simulink model "TL1_cs"  (R2019a)
settings: Solver=FixedStepDiscrete  StartTime=0.0  StopTime=40  FixedStep=1/300  RelTol=1e-3
PreLoadFcn:
  | mbxruntime.callbacks.PreLoadFcn(bdroot);
  | check_NUTS_defined
  | model_closed = 0;
  | assignin('base',['model_closed_' bdroot],false);
PostLoadFcn:
  | mbxruntime.callbacks.PostLoadFcn(bdroot);
InitFcn:
  | mbxruntime.callbacks.InitFcn(bdroot);
StartFcn:
  | mbxruntime.callbacks.StartFcn(bdroot);
StopFcn:
  | mbxruntime.callbacks.StopFcn(bdroot);;
  | 
model workspace: external: MAT-File .\TL1_cs_hws.mat (data not in the file)
undefined symbols (not defined in the file): AngularVelocity, Clock_, Data, Data_SL_Info, DiscIntNeverNeededParam, Encoding, Encoding_SL_Info, Header, Height, InitImageOutputDir, LinearAcceleration, mbxruntime, Orientation, Pose, Poses, Poses_SL_Info, Position, Step, tabledata, Twist, Width
libraries: robotlib x24, simulink_extras x16, PreScanSimulinkLibrary x4, dspindex x4, robotcorelib x2, visionconversions x2, visionsinks x2, sharedtransform x1
(part 3 of 4)

== system TL1_cs/BMW_X5_SUV_1/Subsystem2 ==
  In1 : Inport
  In2 : Inport  Port=2
  In3 : Inport  Port=3
  In4 : Inport  Port=4
  In5 : Inport  Port=5
  Matrix Concatenate5 : Concatenate  NumInputs=4  Mode=Multidimensional array  ConcatenateDimension=2
  Reshape{1..4} (4 alike) : Reshape
  Rotate over Z : Subsystem
  Spherical to cartesian : Subsystem
  Out1 : Outport
  wires:
  In5/1 -> Reshape3/1
  Reshape4/1 -> Spherical to cartesian/1(In1)
  In1/1 -> Rotate over Z/1(In1)
  Reshape1/1 -> Spherical to cartesian/2(In2)
  Spherical to cartesian/1(Out1) -> Rotate over Z/2(In2)
  Reshape2/1 -> Spherical to cartesian/3(In3)
  Spherical to cartesian/2(Out2) -> Rotate over Z/3(In3)
  In3/1 -> Reshape1/1
  Rotate over Z/2(Out2) -> Matrix Concatenate5/2
  Spherical to cartesian/3(Out3) -> Matrix Concatenate5/3
  Reshape3/1 -> Matrix Concatenate5/4
  Rotate over Z/1(Out1) -> Matrix Concatenate5/1
  Matrix Concatenate5/1 -> Out1/1
  In2/1 -> Reshape4/1
  In4/1 -> Reshape2/1

== system TL1_cs/BMW_X5_SUV_1/Subsystem3 ==
  In1 : Inport
  In2 : Inport  Port=2
  In3 : Inport  Port=3
  In4 : Inport  Port=4
  In5 : Inport  Port=5
  Matrix Concatenate5 : Concatenate  NumInputs=4  Mode=Multidimensional array  ConcatenateDimension=2
  Reshape{1..4} (4 alike) : Reshape
  Rotate over Z : Subsystem
  Spherical to cartesian : Subsystem
  Out1 : Outport
  wires:
  In5/1 -> Reshape3/1
  Reshape4/1 -> Spherical to cartesian/1(In1)
  In1/1 -> Rotate over Z/1(In1)
  Reshape1/1 -> Spherical to cartesian/2(In2)
  Spherical to cartesian/1(Out1) -> Rotate over Z/2(In2)
  Reshape2/1 -> Spherical to cartesian/3(In3)
  Spherical to cartesian/2(Out2) -> Rotate over Z/3(In3)
  In3/1 -> Reshape1/1
  Rotate over Z/2(Out2) -> Matrix Concatenate5/2
  Spherical to cartesian/3(Out3) -> Matrix Concatenate5/3
  Reshape3/1 -> Matrix Concatenate5/4
  Rotate over Z/1(Out1) -> Matrix Concatenate5/1
  Matrix Concatenate5/1 -> Out1/1
  In2/1 -> Reshape4/1
  In4/1 -> Reshape2/1

== system TL1_cs/BMW_X5_SUV_1/camera_CM_Demux ==
  In1 : Inport
  Selector : Selector  NumberOfDimensions=2  InputPortWidth=3  IndexOptions=Index vector (dialog),Index vector (dialog)  Indices=-1,1:hres  OutputSizes=1,1
  Selector1 : Selector  NumberOfDimensions=2  InputPortWidth=3  IndexOptions=Index vector (dialog),Index vector (dialog)  Indices=-1,hres+1:hres*2  OutputSizes=1,1
  Selector2 : Selector  NumberOfDimensions=2  InputPortWidth=3  IndexOptions=Index vector (dialog),Index vector (dialog)  Indices=-1,hres*2+1:hres*3  OutputSizes=1,1
  R : Outport
  G : Outport  Port=2
  B : Outport  Port=3
  wires:
  In1/1 -> Selector1/1, Selector/1, Selector2/1
  Selector/1 -> R/1
  Selector1/1 -> G/1
  Selector2/1 -> B/1

== system TL1_cs/BMW_X5_SUV_1/clock ==
  note: Nanoseconds
  In1 : Inport
  Enable : EnablePort
  Blank Message3 : robotlib/Blank Message  messageClass=Message  entityType=rosgraph_msgs/Clock  messageType=rosgraph_msgs/Clock  SampleTime=inf
      settings: SourceProductBaseCode=RO
  Bus Assignment : BusAssignment  AssignedSignals=Clock_.Sec,Clock_.Nsec
  Constant2 : Constant  Value=1000000000
  Floor : Rounding  Operator=fix
  Product : Product
  Publish3 : robotlib/Publish  topicSource=Specify your own  topic=/clock  messageType=rosgraph_msgs/Clock  messageQueueLength=1
      settings: SourceProductBaseCode=RO
  Subtract : Sum  Inputs=+-
  wires:
  Constant2/1 -> Product/2
  Product/1 -> Bus Assignment/3
  Subtract/1 -> Product/1
  Bus Assignment/1 -> Publish3/1
  Blank Message3/1 -> Bus Assignment/1
  Floor/1 -> Bus Assignment/2, Subtract/2
  In1/1 -> Floor/1, Subtract/1

== system TL1_cs/BMW_X5_SUV_1/current_velocity ==
  In1 : Inport
  In2 : Inport  Port=2
  Enable : EnablePort
  Add5 : Sum
  Assignment2 : Assignment  OutputInitialize=Specify size for each dimension in table  DiagnosticForDimensions=Warning  IndexOptions=Starting index (dialog)  Indices=1  OutputSizes=1000
  Blank Message6 : robotlib/Blank Message  messageClass=Message  entityType=geometry_msgs/TwistStamped  messageType=geometry_msgs/TwistStamped  SampleTime=inf
      settings: SourceProductBaseCode=RO
  Bus Assignment5 : BusAssignment  AssignedSignals=Header.Seq,Header.FrameId,Header.FrameId_SL_Info.CurrentLength,Twist.Linear.X,Twist.Linear.Y,Twist.Linear.Z,Twist.Angular.X,Twist.Angular.Y,Twist.Angular.Z
  Bus Selector2 : BusSelector  OutputSignals=Header.FrameId
  Constant{18..21} (4 alike) : Constant  Value=0
  Constant24 : Constant  OutDataTypeStr=uint32
  Constant25 : Constant  Value=uint8(['/base_link'])
  Degrees to Radians3 : simulink_extras/Transformations/Degrees to Radians
  Memory2 : Memory  InheritSampleTime=on
  Publish4 : robotlib/Publish  topicSource=Select from ROS network  topic=/current_velocity  messageType=geometry_msgs/TwistStamped  messageQueueLength=1
      settings: SourceProductBaseCode=RO
  Width5 : Width  DataType=uint32
  wires:
  In2/1 -> Degrees to Radians3/1
  In1/1 -> Bus Assignment5/5
  Bus Assignment5/1 -> Publish4/1
  Constant21/1 -> Bus Assignment5/9
  Blank Message6/1 -> Bus Assignment5/1, Bus Selector2/1
  Constant18/1 -> Bus Assignment5/6
  Add5/1 -> Memory2/1, Bus Assignment5/2
  Bus Selector2/1 -> Assignment2/1  "<FrameId>"
  Constant20/1 -> Bus Assignment5/8
  Width5/1 -> Bus Assignment5/4
  Constant24/1 -> Add5/2
  Constant19/1 -> Bus Assignment5/7
  Degrees to Radians3/1 -> Bus Assignment5/10
  Memory2/1 -> Add5/1
  Assignment2/1 -> Bus Assignment5/3
  Constant25/1 -> Width5/1, Assignment2/2

== system TL1_cs/BMW_X5_SUV_1/gnss_pose_simulink ==
  In1 : Inport
  Enable : EnablePort
  Blank Message4 : robotlib/Blank Message  messageClass=Message  entityType=geometry_msgs/Pose  messageType=geometry_msgs/Pose  SampleTime=inf
      settings: SourceProductBaseCode=RO
  Bus Assignment3 : BusAssignment  AssignedSignals=Position.X,Position.Y,Position.Z,Orientation.W,Orientation.X,Orientation.Y,Orientation.Z
  Demux : Demux  Outputs=7
  Publish2 : robotlib/Publish  topicSource=Specify your own  topic=/gnss_pose_simulink  messageType=geometry_msgs/Pose  messageQueueLength=1
      settings: SourceProductBaseCode=RO
  wires:
  Demux/1 -> Bus Assignment3/2
  Demux/6 -> Bus Assignment3/7
  In1/1 -> Demux/1
  Demux/2 -> Bus Assignment3/3
  Demux/7 -> Bus Assignment3/8
  Demux/5 -> Bus Assignment3/6
  Demux/3 -> Bus Assignment3/4
  Demux/4 -> Bus Assignment3/5
  Blank Message4/1 -> Bus Assignment3/1
  Bus Assignment3/1 -> Publish2/1

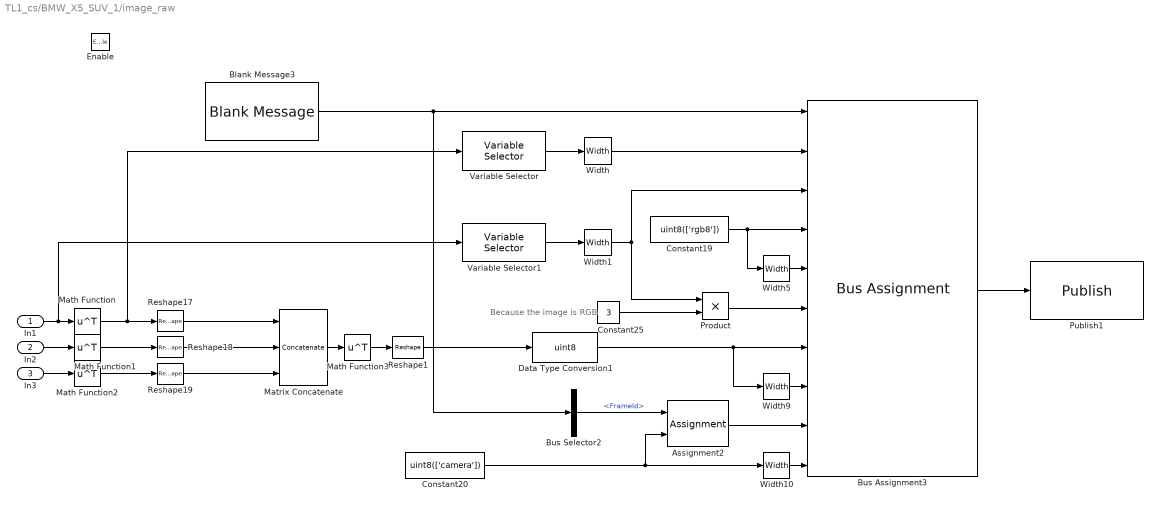
== system TL1_cs/BMW_X5_SUV_1/image_raw ==
  note: Because the image is RGB
  In1 : Inport
  In2 : Inport  Port=2
  In3 : Inport  Port=3
  Enable : EnablePort
  Assignment2 : Assignment  OutputInitialize=Specify size for each dimension in table  DiagnosticForDimensions=Warning  IndexOptions=Starting index (dialog)  Indices=1  OutputSizes=1000
  Blank Message3 : robotlib/Blank Message  messageClass=Message  entityType=sensor_msgs/Image  messageType=sensor_msgs/Image  SampleTime=inf
      settings: SourceProductBaseCode=RO
  Bus Assignment3 : BusAssignment  AssignedSignals=Height,Width,Encoding,Encoding_SL_Info.CurrentLength,Step,Data,Data_SL_Info.CurrentLength,Header.FrameId,Header.FrameId_SL_Info.CurrentLength
  Bus Selector2 : BusSelector  OutputSignals=Header.FrameId
  Constant19 : Constant  Value=uint8(['rgb8'])
  Constant20 : Constant  Value=uint8(['camera'])
  Constant25 : Constant  Value=3  OutDataTypeStr=Inherit: Inherit via back propagation
  Data Type Conversion1 : DataTypeConversion  OutDataTypeStr=uint8
  Math Function{,1..3} (4 alike) : Math  Operator=transpose  SaturateOnIntegerOverflow=on
  Matrix Concatenate : Concatenate  NumInputs=3  Mode=Multidimensional array  ConcatenateDimension=2
  Product : Product  OutDataTypeStr=uint32
  Publish1 : robotlib/Publish  topicSource=Specify your own  topic=/image_raw  messageType=sensor_msgs/Image  messageQueueLength=1
      settings: SourceProductBaseCode=RO
  Reshape{1,17..19} (4 alike) : Reshape
  Variable Selector : dspindex/Variable Selector  NumInputs=1  rowsOrCols=Rows  IdxMode=Fixed  Elements=[1]  ZerOneIdxMode=One-based  errmode=Clip Index  FillMode=on  FillValues=0
  Variable Selector1 : dspindex/Variable Selector  NumInputs=1  rowsOrCols=Rows  IdxMode=Fixed  Elements=[1]  ZerOneIdxMode=One-based  errmode=Clip Index  FillMode=on  FillValues=0
  Width : Width
  Width1 : Width
  Width10 : Width  DataType=uint32
  Width5 : Width  DataType=uint32
  Width9 : Width  DataType=uint32
  wires:
  Variable Selector1/1 -> Width1/1
  Variable Selector/1 -> Width/1
  Math Function3/1 -> Reshape1/1
  Matrix Concatenate/1 -> Math Function3/1
  Reshape1/1 -> Data Type Conversion1/1
  In1/1 -> Math Function/1, Variable Selector1/1
  In2/1 -> Math Function1/1
  In3/1 -> Math Function2/1
  Blank Message3/1 -> Bus Assignment3/1, Bus Selector2/1
  Math Function1/1 -> Reshape18/1
  Width1/1 -> Product/1, Bus Assignment3/3
  Constant20/1 -> Width10/1, Assignment2/2
  Math Function2/1 -> Reshape19/1
  Width10/1 -> Bus Assignment3/10
  Reshape17/1 -> Matrix Concatenate/1
  Width5/1 -> Bus Assignment3/5
  Reshape18/1 -> Matrix Concatenate/2
  Constant19/1 -> Bus Assignment3/4, Width5/1
  Bus Assignment3/1 -> Publish1/1
  Assignment2/1 -> Bus Assignment3/9
  Product/1 -> Bus Assignment3/6
  Bus Selector2/1 -> Assignment2/1  "<FrameId>"
  Width9/1 -> Bus Assignment3/8
  Width/1 -> Bus Assignment3/2
  Constant25/1 -> Product/2
  Math Function/1 -> Reshape17/1, Variable Selector/1
  Data Type Conversion1/1 -> Bus Assignment3/7, Width9/1
  Reshape19/1 -> Matrix Concatenate/3

== system TL1_cs/BMW_X5_SUV_1/move_base_simple//goal ==
  In1 : Inport
  Enable : EnablePort
  Add4 : Sum
  Assignment4 : Assignment  OutputInitialize=Specify size for each dimension in table  DiagnosticForDimensions=Warning  IndexOptions=Starting index (dialog)  Indices=1  OutputSizes=1000
  Blank Message5 : robotlib/Blank Message  messageClass=Message  entityType=geometry_msgs/PoseStamped  messageType=geometry_msgs/PoseStamped  SampleTime=inf
      settings: SourceProductBaseCode=RO
  Bus Assignment4 : BusAssignment  AssignedSignals=Header.Seq,Header.FrameId,Header.FrameId_SL_Info.CurrentLength,Pose.Position.X,Pose.Position.Y,Pose.Position.Z,Pose.Orientation.W,Pose.Orientation.X,Pose.Orientation.Y,Pose.Orientation.Z
  Bus Selector3 : BusSelector  OutputSignals=Header.FrameId
  Constant8 : Constant  OutDataTypeStr=uint32
  Constant9 : Constant  Value=uint8(['world'])
  Demux : Demux  Outputs=7
  Memory1 : Memory  InheritSampleTime=on
  Publish1 : robotlib/Publish  topicSource=Select from ROS network  topic=/move_base_simple/goal  messageType=geometry_msgs/PoseStamped  messageQueueLength=1
      settings: SourceProductBaseCode=RO
  Width4 : Width  DataType=uint32
  wires:
  Demux/7 -> Bus Assignment4/11
  Demux/6 -> Bus Assignment4/10
  Demux/5 -> Bus Assignment4/9
  Demux/4 -> Bus Assignment4/8
  Demux/3 -> Bus Assignment4/7
  Demux/2 -> Bus Assignment4/6
  Demux/1 -> Bus Assignment4/5
  In1/1 -> Demux/1
  Width4/1 -> Bus Assignment4/4
  Memory1/1 -> Add4/1
  Constant9/1 -> Width4/1, Assignment4/2
  Constant8/1 -> Add4/2
  Bus Assignment4/1 -> Publish1/1
  Bus Selector3/1 -> Assignment4/1  "<FrameId>"
  Assignment4/1 -> Bus Assignment4/3
  Add4/1 -> Memory1/1, Bus Assignment4/2
  Blank Message5/1 -> Bus Assignment4/1, Bus Selector3/1

== system TL1_cs/BMW_X5_SUV_1/points_raw_float32 ==
  In1 : Inport
  In5 : Inport  Port=2
  In9 : Inport  Port=3
  In13 : Inport  Port=4
  Enable : EnablePort
  Blank Message3 : robotlib/Blank Message  messageClass=Message  entityType=std_msgs/Float32MultiArray  messageType=std_msgs/Float32MultiArray  SampleTime=inf
      settings: SourceProductBaseCode=RO
  Bus Assignment3 : BusAssignment  AssignedSignals=Data,Data_SL_Info.CurrentLength
  Data Type Conversion2 : DataTypeConversion  OutDataTypeStr=single
  Math Function1 : Math  Operator=transpose  SaturateOnIntegerOverflow=on
  Matrix Concatenate5 : Concatenate  NumInputs=4  Mode=Multidimensional array
  Publish1 : robotlib/Publish  topicSource=Specify your own  topic=/points_raw_float32  messageType=std_msgs/Float32MultiArray  messageQueueLength=1
      settings: SourceProductBaseCode=RO
  Reshape17 : Reshape
  Width5 : Width  DataType=uint32
  wires:
  Width5/1 -> Bus Assignment3/3
  Matrix Concatenate5/1 -> Math Function1/1
  Reshape17/1 -> Data Type Conversion2/1
  Bus Assignment3/1 -> Publish1/1
  Blank Message3/1 -> Bus Assignment3/1
  Data Type Conversion2/1 -> Width5/1, Bus Assignment3/2
  Math Function1/1 -> Reshape17/1
  In1/1 -> Matrix Concatenate5/1
  In5/1 -> Matrix Concatenate5/2
  In9/1 -> Matrix Concatenate5/3
  In13/1 -> Matrix Concatenate5/4

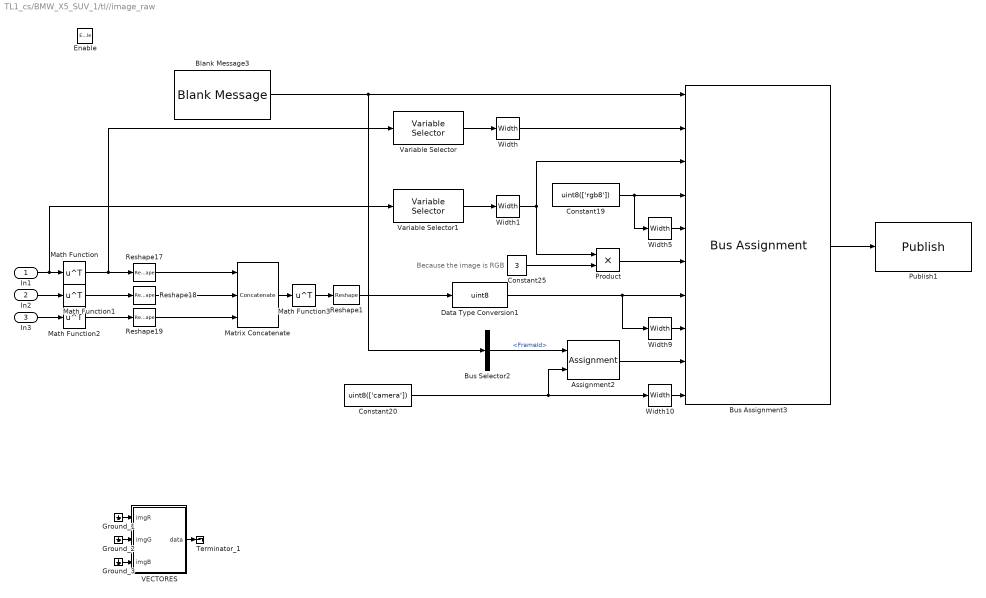
== system TL1_cs/BMW_X5_SUV_1/tl//image_raw ==
  note: Because the image is RGB
  In1 : Inport
  In2 : Inport  Port=2
  In3 : Inport  Port=3
  Enable : EnablePort
  Assignment2 : Assignment  OutputInitialize=Specify size for each dimension in table  DiagnosticForDimensions=Warning  IndexOptions=Starting index (dialog)  Indices=1  OutputSizes=1000
  Blank Message3 : robotlib/Blank Message  messageClass=Message  entityType=sensor_msgs/Image  messageType=sensor_msgs/Image  SampleTime=inf
      settings: SourceProductBaseCode=RO
  Bus Assignment3 : BusAssignment  AssignedSignals=Height,Width,Encoding,Encoding_SL_Info.CurrentLength,Step,Data,Data_SL_Info.CurrentLength,Header.FrameId,Header.FrameId_SL_Info.CurrentLength
  Bus Selector2 : BusSelector  OutputSignals=Header.FrameId
  Constant19 : Constant  Value=uint8(['rgb8'])
  Constant20 : Constant  Value=uint8(['camera'])
  Constant25 : Constant  Value=3  OutDataTypeStr=Inherit: Inherit via back propagation
  Data Type Conversion1 : DataTypeConversion  OutDataTypeStr=uint8
  Ground_1 : Ground
  Ground_2 : Ground
  Ground_3 : Ground
  Math Function{,1..3} (4 alike) : Math  Operator=transpose  SaturateOnIntegerOverflow=on
  Matrix Concatenate : Concatenate  NumInputs=3  Mode=Multidimensional array  ConcatenateDimension=2
  Product : Product  OutDataTypeStr=uint32
  Publish1 : robotlib/Publish  topicSource=Specify your own  topic=/tl/image_raw  messageType=sensor_msgs/Image  messageQueueLength=1
      settings: SourceProductBaseCode=RO
  Reshape{1,17..19} (4 alike) : Reshape
  Terminator_1 : Terminator
  VECTORES : MATLAB Function  TreatAsAtomicUnit=on
  Variable Selector : dspindex/Variable Selector  NumInputs=1  rowsOrCols=Rows  IdxMode=Fixed  Elements=[1]  ZerOneIdxMode=One-based  errmode=Clip Index  FillMode=on  FillValues=0
  Variable Selector1 : dspindex/Variable Selector  NumInputs=1  rowsOrCols=Rows  IdxMode=Fixed  Elements=[1]  ZerOneIdxMode=One-based  errmode=Clip Index  FillMode=on  FillValues=0
  Width : Width
  Width1 : Width
  Width10 : Width  DataType=uint32
  Width5 : Width  DataType=uint32
  Width9 : Width  DataType=uint32
  wires:
  VECTORES/1(data) -> Terminator_1/1
  Ground_3/1 -> VECTORES/3(imgB)
  Ground_2/1 -> VECTORES/2(imgG)
  Ground_1/1 -> VECTORES/1(imgR)
  Variable Selector1/1 -> Width1/1
  Variable Selector/1 -> Width/1
  Math Function3/1 -> Reshape1/1
  Matrix Concatenate/1 -> Math Function3/1
  Reshape1/1 -> Data Type Conversion1/1
  In1/1 -> Math Function/1, Variable Selector1/1
  In2/1 -> Math Function1/1
  In3/1 -> Math Function2/1
  Blank Message3/1 -> Bus Assignment3/1, Bus Selector2/1
  Math Function1/1 -> Reshape18/1
  Width1/1 -> Product/1, Bus Assignment3/3
  Constant20/1 -> Width10/1, Assignment2/2
  Math Function2/1 -> Reshape19/1
  Width10/1 -> Bus Assignment3/10
  Reshape17/1 -> Matrix Concatenate/1
  Width5/1 -> Bus Assignment3/5
  Reshape18/1 -> Matrix Concatenate/2
  Constant19/1 -> Bus Assignment3/4, Width5/1
  Bus Assignment3/1 -> Publish1/1
  Assignment2/1 -> Bus Assignment3/9
  Product/1 -> Bus Assignment3/6
  Bus Selector2/1 -> Assignment2/1  "<FrameId>"
  Width9/1 -> Bus Assignment3/8
  Width/1 -> Bus Assignment3/2
  Constant25/1 -> Product/2
  Math Function/1 -> Reshape17/1, Variable Selector/1
  Data Type Conversion1/1 -> Bus Assignment3/7, Width9/1
  Reshape19/1 -> Matrix Concatenate/3

== system TL1_cs/BMW_X5_SUV_1/tl_camera_CM_Demux ==
  In1 : Inport
  Selector : Selector  NumberOfDimensions=2  InputPortWidth=3  IndexOptions=Index vector (dialog),Index vector (dialog)  Indices=-1,1:hres  OutputSizes=1,1
  Selector1 : Selector  NumberOfDimensions=2  InputPortWidth=3  IndexOptions=Index vector (dialog),Index vector (dialog)  Indices=-1,hres+1:hres*2  OutputSizes=1,1
  Selector2 : Selector  NumberOfDimensions=2  InputPortWidth=3  IndexOptions=Index vector (dialog),Index vector (dialog)  Indices=-1,hres*2+1:hres*3  OutputSizes=1,1
  R : Outport
  G : Outport  Port=2
  B : Outport  Port=3
  wires:
  In1/1 -> Selector1/1, Selector/1, Selector2/1
  Selector/1 -> R/1
  Selector1/1 -> G/1
  Selector2/1 -> B/1

== system TL1_cs/BMW_X5_SUV_1/tonemap ==
  In1 : Inport
  Constant : Constant  Value=255
  Data Type Conversion : DataTypeConversion  OutDataTypeStr=uint8
  Product : Product
  Square Root : Sqrt  SaturateOnIntegerOverflow=on
  Out1 : Outport
  wires:
  In1/1 -> Square Root/1
  Square Root/1 -> Product/1
  Product/1 -> Data Type Conversion/1
  Constant/1 -> Product/2
  Data Type Conversion/1 -> Out1/1

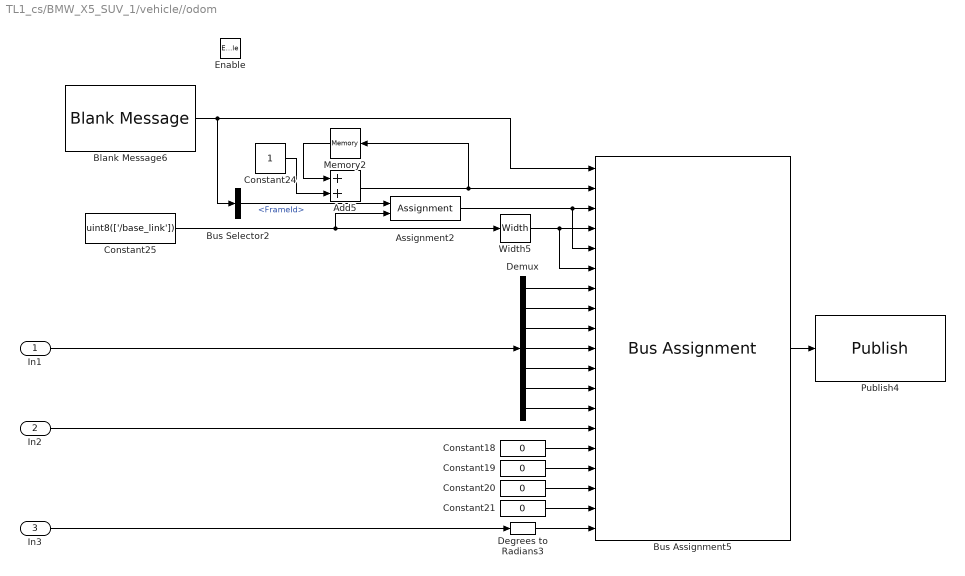
== system TL1_cs/BMW_X5_SUV_1/vehicle//odom ==
  In1 : Inport
  In2 : Inport  Port=2
  In3 : Inport  Port=3
  Enable : EnablePort
  Add5 : Sum
  Assignment2 : Assignment  OutputInitialize=Specify size for each dimension in table  DiagnosticForDimensions=Warning  IndexOptions=Starting index (dialog)  Indices=1  OutputSizes=1000
  Blank Message6 : robotlib/Blank Message  messageClass=Message  entityType=nav_msgs/Odometry  messageType=nav_msgs/Odometry  SampleTime=inf
      settings: SourceProductBaseCode=RO
  Bus Assignment5 : BusAssignment  AssignedSignals=Header.Seq,Header.FrameId,Header.FrameId_SL_Info.CurrentLength,ChildFrameId,ChildFrameId_SL_Info.CurrentLength,Pose.Pose.Position.X,Pose.Pose.Position.Y,Pose.Pose.Position.Z,Pose.Pose.Orientation.W,Pose.Pose.Orientation.X,Pose.Pose.Orientation.Y,Pose.Pose.Orientation.Z,Twist.Twist.Linear.X,Twist.Twist.Linear.Y,Twist.Twist.Linear.Z,Twist.Twist.Angular.X,Twist.Twist.Angular.Y,Twist.Twist.Angular.Z
  Bus Selector2 : BusSelector  OutputSignals=Header.FrameId
  Constant{18..21} (4 alike) : Constant  Value=0
  Constant24 : Constant  OutDataTypeStr=uint32
  Constant25 : Constant  Value=uint8(['/base_link'])
  Degrees to Radians3 : simulink_extras/Transformations/Degrees to Radians
  Demux : Demux  Outputs=7
  Memory2 : Memory  InheritSampleTime=on
  Publish4 : robotlib/Publish  topicSource=Specify your own  topic=/vehicle/odom  messageType=nav_msgs/Odometry  messageQueueLength=1
      settings: SourceProductBaseCode=RO
  Width5 : Width  DataType=uint32
  wires:
  Demux/1 -> Bus Assignment5/7
  Demux/5 -> Bus Assignment5/11
  Demux/4 -> Bus Assignment5/10
  In1/1 -> Demux/1
  Demux/6 -> Bus Assignment5/12
  Demux/7 -> Bus Assignment5/13
  Demux/2 -> Bus Assignment5/8
  Demux/3 -> Bus Assignment5/9
  In2/1 -> Bus Assignment5/14
  Constant21/1 -> Bus Assignment5/18
  Constant19/1 -> Bus Assignment5/16
  Constant20/1 -> Bus Assignment5/17
  Degrees to Radians3/1 -> Bus Assignment5/19
  Constant18/1 -> Bus Assignment5/15
  In3/1 -> Degrees to Radians3/1
  Bus Assignment5/1 -> Publish4/1
  Blank Message6/1 -> Bus Assignment5/1, Bus Selector2/1
  Add5/1 -> Memory2/1, Bus Assignment5/2
  Bus Selector2/1 -> Assignment2/1  "<FrameId>"
  Width5/1 -> Bus Assignment5/4, Bus Assignment5/6
  Constant24/1 -> Add5/2
  Memory2/1 -> Add5/1
  Assignment2/1 -> Bus Assignment5/3, Bus Assignment5/5
  Constant25/1 -> Width5/1, Assignment2/2

== system TL1_cs/Ford_Fiesta_Hatchback_1/AIR_1_Demux ==
  AIR : Inport
  Activate_Switch : Subsystem
      mask Display: text(5,10,'')
  Bus Selector : BusSelector  OutputSignals=DATA.Range,DATA.Azimuth,DATA.Elevation,DATA.ID,DATA.Velocity,DATA.Heading
  Data Type Conversion : DataTypeConversion  OutDataTypeStr=double
  For Iterator : ForIterator  ResetStates=reset  IterationLimit=detectableObjects
  Selector : Selector  InputPortWidth=detectableObjects  IndexOptions=Index vector (port)  Indices=[1 3]  OutputSizes=1
  Signal2ArrayOfSignals1 : Subsystem  mask{VECTORLENGTH=detectableObjects}
      mask prompts: VECTORLENGTH "Length of vector"
  Signal2ArrayOfSignals2 : Subsystem  mask{VECTORLENGTH=detectableObjects}
      mask prompts: VECTORLENGTH "Length of vector"
  Signal2ArrayOfSignals3 : Subsystem  mask{VECTORLENGTH=detectableObjects}
      mask prompts: VECTORLENGTH "Length of vector"
  Signal2ArrayOfSignals4 : Subsystem  mask{VECTORLENGTH=detectableObjects}
      mask prompts: VECTORLENGTH "Length of vector"
  Signal2ArrayOfSignals5 : Subsystem  mask{VECTORLENGTH=detectableObjects}
      mask prompts: VECTORLENGTH "Length of vector"
  Signal2ArrayOfSignals6 : Subsystem  mask{VECTORLENGTH=detectableObjects}
      mask prompts: VECTORLENGTH "Length of vector"
  Range [m] : Outport
  Azimuth [deg] : Outport  Port=2
  Elevation [deg] : Outport  Port=3
  ID [-] : Outport  Port=4
  Velocity [m/s] : Outport  Port=5
  Heading [deg] : Outport  Port=6
  wires:
  Data Type Conversion/1 -> ID [-]/1
  Bus Selector/6 -> Signal2ArrayOfSignals6/2(Element)  "<Heading>"
  Signal2ArrayOfSignals6/1(ArrayofElements) -> Activate_Switch/2(Heading)
  Bus Selector/5 -> Signal2ArrayOfSignals5/2(Element)  "<Velocity>"
  Signal2ArrayOfSignals5/1(ArrayofElements) -> Velocity [m/s]/1
  Bus Selector/4 -> Signal2ArrayOfSignals4/2(Element)  "<ID>"
  Signal2ArrayOfSignals4/1(ArrayofElements) -> Data Type Conversion/1, Activate_Switch/1(BeamID)
  Bus Selector/3 -> Signal2ArrayOfSignals3/2(Element)  "<Elevation>"
  Signal2ArrayOfSignals3/1(ArrayofElements) -> Elevation [deg]/1
  Bus Selector/2 -> Signal2ArrayOfSignals1/2(Element)  "<Azimuth>"
  Signal2ArrayOfSignals1/1(ArrayofElements) -> Azimuth [deg]/1
  Signal2ArrayOfSignals2/1(ArrayofElements) -> Range [m]/1
  Bus Selector/1 -> Signal2ArrayOfSignals2/2(Element)  "<Range>"
  Selector/1 -> Bus Selector/1
  For Iterator/1 -> Signal2ArrayOfSignals6/1(LoopIndex), Signal2ArrayOfSignals5/1(LoopIndex), Signal2ArrayOfSignals4/1(LoopIndex), Signal2ArrayOfSignals3/1(LoopIndex), Signal2ArrayOfSignals1/1(LoopIndex), Signal2ArrayOfSignals2/1(LoopIndex), Selector/2
  AIR/1 -> Selector/1
  Activate_Switch/1(On/Off) -> Heading [deg]/1

== system TL1_cs/Ford_Fiesta_Hatchback_1/Car_Pos_and_Orient ==
  In1 : Inport
  In2 : Inport  Port=2
  In3 : Inport  Port=3
  In4 : Inport  Port=4
  In5 : Inport  Port=5
  In6 : Inport  Port=6
  Data Type Conversion : DataTypeConversion
  Data Type Conversion1 : DataTypeConversion
  Data Type Conversion2 : DataTypeConversion
  Degrees to Radians1 : simulink_extras/Transformations/Degrees to Radians
  Degrees to Radians2 : simulink_extras/Transformations/Degrees to Radians
  Degrees to Radians5 : simulink_extras/Transformations/Degrees to Radians
  Mux : Mux
  Rotation Angles to Quaternions : sharedtransform/Rotation Angles to Quaternions  rotationOrder=XYZ  aMode=aMode
      settings: SourceProductName=Aerospace Blockset  SourceProductBaseCode=AE
  Vector Concatenate2 : Concatenate  NumInputs=3
  Out1 : Outport
  wires:
  Mux/1 -> Out1/1
  Rotation Angles to Quaternions/1 -> Mux/4
  Data Type Conversion2/1 -> Mux/3
  Data Type Conversion1/1 -> Mux/2
  Data Type Conversion/1 -> Mux/1
  In6/1 -> Degrees to Radians2/1
  In5/1 -> Degrees to Radians1/1
  In4/1 -> Degrees to Radians5/1
  In3/1 -> Data Type Conversion2/1
  In2/1 -> Data Type Conversion1/1
  In1/1 -> Data Type Conversion/1
  Degrees to Radians2/1 -> Vector Concatenate2/3
  Vector Concatenate2/1 -> Rotation Angles to Quaternions/1
  Degrees to Radians5/1 -> Vector Concatenate2/1
  Degrees to Radians1/1 -> Vector Concatenate2/2

== system TL1_cs/Ford_Fiesta_Hatchback_1/Dynamics_Empty ==
  note: For state mode 'Dynamic' positions
      | are not taken into account, as they
      | are computed by integrating velocity.
      | Click annotation for Help.
  Ground_{1..8} (8 alike) : Ground
  Memory2 : Memory  InheritSampleTime=on
  MinMax : MinMax  Function=max  Inputs=2
  MuxState : Subsystem  Tag=mux/State  mask(Empty Dynamics State Block){positioningmode=off, TimeStep=1/300}
      mask prompts: positioningmode "Positioning Mode"; TimeStep "Auto Assigned: Time Step [s]"
      mask help:
      | Build the state of an actor based on user input.
      | The user can either use positioning mode or dynamics mode.
      | - When using positioning mode the position and orientation of the actor are set directly based on the input. Expected input is relative to the initial position and orientation of the actor. It's also possible to specify the velocity of the actor, though this input isn't used, only passed on.
      | - When using dynamics mode the position input is ignored. Expected input is velocity and orientation. The velocity is relative the current orientation of the actor, while orientation is relative to its initial orientation. The position of the actor is calculated based on the velocity and orientation given.
      settings: DeleteFcn=PreScanBlockDeleteFcn;
  STATE_Ford_Fiesta_Hatchback_1 : Subsystem  Tag=mux/StatePort  Priority=0  LoadFcn=load PrescanStateActuatorData  mask(PreScan Sink Block: State){x0=-29.0644, y0=3.2788, z0=0.53, Roll0=0, Pitch0=0, Yaw0=270.6587, TimeStep=1/300}
      mask prompts: x0 "Ini x-position VEHICLE wrt GLOBAL axis system [m]"; y0 "Ini y-position VEHICLE wrt GLOBAL axis system [m]"; z0 "Ini z-position VEHICLE wrt GLOBAL axis system [m]"; Roll0 "Ini roll-angle BODY wrt VEHICLE axis system [deg]"; Pitch0 "Ini pitch-angle BODY wrt VEHICLE axis system [deg]"; Yaw0 "Ini yaw-angle VEHICLE wrt GLOBAL axis system [deg]"; TimeStep "Auto-Assigned: Upload Period [s]"
      mask help:
      | The Actor State contains a vector signal of size (9x1), containing the following signals:
      |
      | -  Position                  (x,y,z)                                     [m]
      | -  Velocity                  (vx,vy,vz)                               [m/s]
      | -  Angles                    (Roll, Pitch, Yaw)                   [rad]
      |
      | The Actor state is defined in the global axis system.
      | The state is superponed on the Initial position defined in the GUI.
      |
      | For more information, please click Help.
      settings: DeleteFcn=PreScanBlockDeleteFcn;
      mask Help: eval('openHelp(222)')
      mask Display: image(imread('State.png'))
  State : Outport  Tag=outport/StateOutport  SampleTime=1/300
  wires:
  [x_speed] -> MinMax/2
  MinMax/1 -> Memory2/1, MuxState/4(dx [m/s])
  Memory2/1 -> MinMax/1
  MuxState/1(state) -> STATE_Ford_Fiesta_Hatchback_1/1(State)
  STATE_Ford_Fiesta_Hatchback_1/1(StateBus) -> State/1
  Ground_1/1 -> MuxState/1(x [m])
  Ground_2/1 -> MuxState/2(y [m])
  Ground_3/1 -> MuxState/3(z [m])
  Ground_4/1 -> MuxState/5(dy [m/s])
  Ground_5/1 -> MuxState/6(dz [m/s])
  Ground_6/1 -> MuxState/7(R [rad])
  Ground_7/1 -> MuxState/8(P [rad])
  Ground_8/1 -> MuxState/9(Y [rad])

== system TL1_cs/Ford_Fiesta_Hatchback_1/SELF_Demux ==
  SELF : Inport  OutDataTypeStr=Bus: PRESCAN_SELFSENSORDATA
  Bus Selector : BusSelector  OutputSignals=PositionX,PositionY,PositionZ,OrientationRoll,OrientationPitch,OrientationYaw,Velocity,Yaw_rate,Lat,Long,Alt
  Demux2 : Demux  Outputs=3
  Gain : Gain  Gain=180/pi
  Gain1 : Gain  Gain=180/pi
  Vector Concatenate1 : Concatenate  NumInputs=3
  compas converter : Subsystem
  x [m] : Outport
  y [m] : Outport  Port=2
  z [m] : Outport  Port=3
  rotx [deg] : Outport  Port=4
  roty [deg] : Outport  Port=5
  rotz [deg] : Outport  Port=6
  GPS lat [deg] : Outport  Port=7
  GPS long [deg] : Outport  Port=8
  GPS alt [m] : Outport  Port=9
  velocity [m/s] : Outport  Port=10
  heading [deg] : Outport  Port=11
  yaw rate [deg/s] : Outport  Port=12
  wires:
  Bus Selector/11 -> GPS alt [m]/1  "<Alt>"
  Bus Selector/10 -> GPS long [deg]/1  "<Long>"
  Bus Selector/9 -> GPS lat [deg]/1  "<Lat>"
  Bus Selector/8 -> Gain1/1  "<Yaw_rate>"
  Bus Selector/7 -> velocity [m/s]/1  "<Velocity>"
  Bus Selector/6 -> compas converter/1(rotz [rad]), Vector Concatenate1/3  "<OrientationYaw>"
  Bus Selector/5 -> Vector Concatenate1/2  "<OrientationPitch>"
  Bus Selector/4 -> Vector Concatenate1/1  "<OrientationRoll>"
  Vector Concatenate1/1 -> Gain/1
  Bus Selector/3 -> z [m]/1  "<PositionZ>"
  Bus Selector/2 -> y [m]/1  "<PositionY>"
  Bus Selector/1 -> x [m]/1  "<PositionX>"
  SELF/1 -> Bus Selector/1
  Gain/1 -> Demux2/1
  Demux2/1 -> rotx [deg]/1
  Demux2/2 -> roty [deg]/1
  Demux2/3 -> rotz [deg]/1
  compas converter/1(heading [deg]) -> heading [deg]/1
  Gain1/1 -> yaw rate [deg/s]/1

== system TL1_cs/Ford_Fiesta_Hatchback_1/message_creator ==
  In1 : Inport
  Blank Message4 : robotlib/Blank Message  messageClass=Message  entityType=geometry_msgs/Pose  messageType=geometry_msgs/Pose  SampleTime=inf
      settings: SourceProductBaseCode=RO
  Bus Assignment3 : BusAssignment  AssignedSignals=Position.X,Position.Y,Position.Z,Orientation.W,Orientation.X,Orientation.Y,Orientation.Z
  Demux : Demux  Outputs=7
  Out1 : Outport
  wires:
  Bus Assignment3/1 -> Out1/1
  Demux/1 -> Bus Assignment3/2
  Demux/6 -> Bus Assignment3/7
  In1/1 -> Demux/1
  Demux/2 -> Bus Assignment3/3
  Demux/7 -> Bus Assignment3/8
  Demux/5 -> Bus Assignment3/6
  Demux/3 -> Bus Assignment3/4
  Demux/4 -> Bus Assignment3/5
  Blank Message4/1 -> Bus Assignment3/1

== system TL1_cs/TrafficLightRoadSideNL_1/VISUCasingLights_Mux ==
  Green [-] : Inport  Tag=inport/Green [-]  SampleTime=1/300  BusOutputAsStruct=on
  Orange [-] : Inport  Tag=inport/Orange [-]  Port=2  SampleTime=1/300  BusOutputAsStruct=on
  Red [-] : Inport  Tag=inport/Red [-]  Port=3  SampleTime=1/300  BusOutputAsStruct=on
  MuxVisuLights : Mux  Inputs=3
  VISUCasingLights_TrafficLightRoadSideNL_1 : Outport  Tag=outport/VisuCasingLights  SampleTime=1/300
  wires:
  MuxVisuLights/1 -> VISUCasingLights_TrafficLightRoadSideNL_1/1
  Green [-]/1 -> MuxVisuLights/1
  Orange [-]/1 -> MuxVisuLights/2
  Red [-]/1 -> MuxVisuLights/3

== system TL1_cs/VISUCasingLights_TrafficLightRoadSideNL_1/Actuator ==
  VISUCasingLights_TrafficLightRoadSideNL_1 : Inport  Tag=inport/VisuCasingLights  SampleTime=1/300  BusOutputAsStruct=on
  DemuxVisuLights : Demux  Outputs=3
  LimiterVisuLights : Saturate  UpperLimit=1  LowerLimit=0
  visu_Green [-] : S-Function  FunctionName=sfun_MaterialColorSelector  Parameters=mbxruntime.parameters.convert(UniqueID), mbxruntime.parameters.convert(ColorsObjectQuery), mbxruntime.parameters.convert(Colors),tabledata, TimeStep  SFunctionDeploymentMode=off  EnableBusSupport=off  mask(PreScan Sink Block: VisuTrafficLight){UniqueID=20538, ColorsObjectQuery=child:name=TrafficLightRoadSideNL_1.Casing.LightGreen, Colors=[5   32   25  255    0   64   50  255    0   64   50  255    0    0    0  255; 0   45   34  255    0   45   34  255    0   45   34  255   30  306  240  255], TimeStep=1/300}
      mask prompts: UniqueID "Parent Unique Identifier"; ColorsObjectQuery "Query for Color Object"; Colors "Matrix of colors"; TimeStep "Simulink time step"
      mask help:
      | The VisuTrafficLight block provides a way to animate traffic lights: switch on and off individual lights.
      |
      | For more information, please click Help.
      mask init:
      | [tabledata] = mbxruntime.parameters.table(UniqueID,ColorsObjectQuery,Colors);
      mask Help: eval('openHelp(731)')
      mask Display: image(imread('TrafficLightCasing.png'))
  visu_Orange [-] : S-Function  FunctionName=sfun_MaterialColorSelector  Parameters=mbxruntime.parameters.convert(UniqueID), mbxruntime.parameters.convert(ColorsObjectQuery), mbxruntime.parameters.convert(Colors),tabledata, TimeStep  SFunctionDeploymentMode=off  EnableBusSupport=off  mask(PreScan Sink Block: VisuTrafficLight){UniqueID=20538, ColorsObjectQuery=child:name=TrafficLightRoadSideNL_1.Casing.LightOrange, Colors=[32   25    5  255   64   48    5  255   64   54    5  255    0    0    0  255; 45   34    0  255   45   34    0  255   45   34    0  255  306  229    5  255], TimeStep=1/300}
      mask prompts: UniqueID "Parent Unique Identifier"; ColorsObjectQuery "Query for Color Object"; Colors "Matrix of colors"; TimeStep "Simulink time step"
      mask help:
      | The VisuTrafficLight block provides a way to animate traffic lights: switch on and off individual lights.
      |
      | For more information, please click Help.
      mask init:
      | [tabledata] = mbxruntime.parameters.table(UniqueID,ColorsObjectQuery,Colors);
      mask Help: eval('openHelp(731)')
      mask Display: image(imread('TrafficLightCasing.png'))
  visu_Red [-] : S-Function  FunctionName=sfun_MaterialColorSelector  Parameters=mbxruntime.parameters.convert(UniqueID), mbxruntime.parameters.convert(ColorsObjectQuery), mbxruntime.parameters.convert(Colors),tabledata, TimeStep  SFunctionDeploymentMode=off  EnableBusSupport=off  mask(PreScan Sink Block: VisuTrafficLight){UniqueID=20538, ColorsObjectQuery=child:name=TrafficLightRoadSideNL_1.Casing.LightRed, Colors=[32    5    5  255   64    5    5  255   64    5    5  255    0    0    0  255; 45    0    0  255   45    0    0  255   45    0    0  255  306   30   30  255], TimeStep=1/300}
      mask prompts: UniqueID "Parent Unique Identifier"; ColorsObjectQuery "Query for Color Object"; Colors "Matrix of colors"; TimeStep "Simulink time step"
      mask help:
      | The VisuTrafficLight block provides a way to animate traffic lights: switch on and off individual lights.
      |
      | For more information, please click Help.
      mask init:
      | [tabledata] = mbxruntime.parameters.table(UniqueID,ColorsObjectQuery,Colors);
      mask Help: eval('openHelp(731)')
      mask Display: image(imread('TrafficLightCasing.png'))
  wires:
  VISUCasingLights_TrafficLightRoadSideNL_1/1 -> LimiterVisuLights/1
  LimiterVisuLights/1 -> DemuxVisuLights/1
  DemuxVisuLights/1 -> visu_Green [-]/1
  DemuxVisuLights/2 -> visu_Orange [-]/1
  DemuxVisuLights/3 -> visu_Red [-]/1

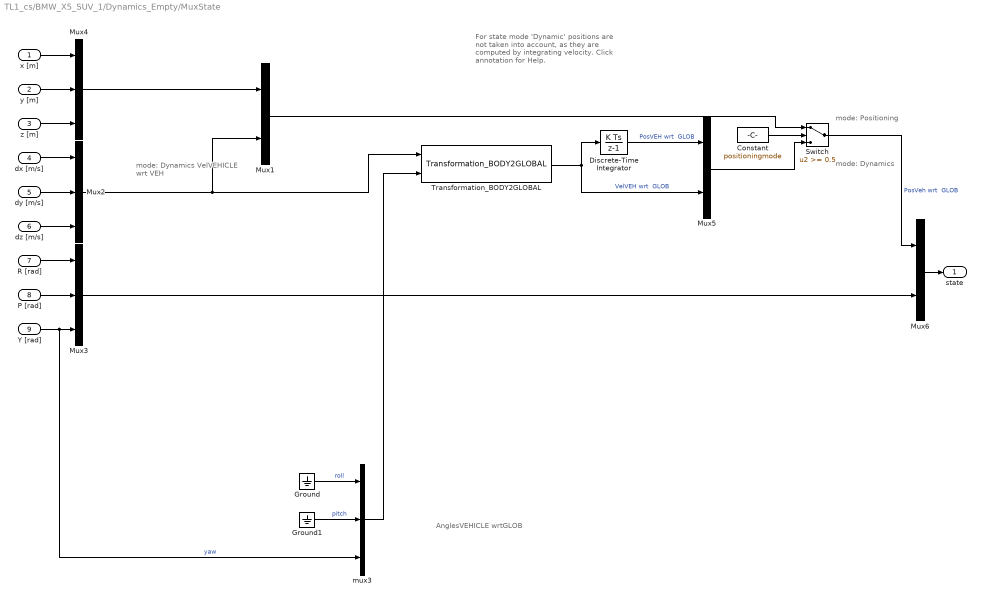
== system TL1_cs/BMW_X5_SUV_1/Dynamics_Empty/MuxState ==
  note: mode: Dynamics
  note: mode: Positioning
  note: mode: Dynamics
      | VelVEHICLE
      | wrt VEH
  note: AnglesVEHICLE
      | wrtGLOB
  note: For state mode 'Dynamic' positions
      | are not taken into account, as they
      | are computed by integrating velocity.
      | Click annotation for Help.
  x [m] : Inport  SampleTime=TimeStep
  y [m] : Inport  Port=2  SampleTime=TimeStep
  z [m] : Inport  Port=3  SampleTime=TimeStep
  dx [m/s] : Inport  Port=4  SampleTime=TimeStep
  dy [m/s] : Inport  Port=5  SampleTime=TimeStep
  dz [m/s] : Inport  Port=6  SampleTime=TimeStep
  R [rad] : Inport  Port=7  SampleTime=TimeStep
  P [rad] : Inport  Port=8  SampleTime=TimeStep
  Y [rad] : Inport  Port=9  SampleTime=TimeStep
  Constant : Constant  DisableCoverage=on  Value=positioningmode
  Discrete-Time Integrator : DiscreteIntegrator  SampleTime=TimeStep  ICPrevOutput=DiscIntNeverNeededParam  ICPrevScaledInput=DiscIntNeverNeededParam
  Ground : Ground
  Ground1 : Ground
  Mux1 : Mux  Inputs=[3 3]
  Mux2 : Mux  Inputs=3
  Mux3 : Mux  Inputs=3
  Mux4 : Mux  Inputs=3
  Mux5 : Mux  Inputs=[3 3]
  Mux6 : Mux  Inputs=[6 3]
  Switch : Switch  Threshold=0.5
  Transformation_BODY2GLOBAL : PreScanSimulinkLibrary/Simple_Vehicle_Dynamics/Chassis/MuxDynState/Transformation_BODY2GLOBAL  SystemSampleTime=-1
  mux3 : Mux  Inputs=3
  state : Outport
  wires:
  Constant/1 -> Switch/2
  Mux6/1 -> state/1
  Mux4/1 -> Mux1/1
  Mux5/1 -> Switch/3
  Mux1/1 -> Switch/1
  Switch/1 -> Mux6/1  "PosVeh wrt  GLOB"
  P [rad]/1 -> Mux3/2
  R [rad]/1 -> Mux3/1
  dz [m/s]/1 -> Mux2/3
  dy [m/s]/1 -> Mux2/2
  dx [m/s]/1 -> Mux2/1
  z [m]/1 -> Mux4/3
  y [m]/1 -> Mux4/2
  x [m]/1 -> Mux4/1
  Ground1/1 -> mux3/2  "pitch"
  Y [rad]/1 -> mux3/3, Mux3/3  "yaw"
  Mux3/1 -> Mux6/2
  Transformation_BODY2GLOBAL/1 -> Discrete-Time Integrator/1, Mux5/2  "VelVEH wrt  GLOB"
  mux3/1 -> Transformation_BODY2GLOBAL/2
  Ground/1 -> mux3/1  "roll"
  Mux2/1 -> Mux1/2, Transformation_BODY2GLOBAL/1
  Discrete-Time Integrator/1 -> Mux5/1  "PosVEH wrt  GLOB"

== system TL1_cs/BMW_X5_SUV_1/Dynamics_Empty/STATE_BMW_X5_SUV_1 ==
  State : Inport  SampleTime=TimeStep
  Bus Creator : BusCreator  Inputs=15  OutDataTypeStr=Bus: PRESCAN_STATEACTUATORDATA  NonVirtualBus=on
  Constant : Constant  Value=0
  Demux : Demux  Outputs=15
  Mux : Mux  Inputs=3
  Mux1 : Mux  Inputs=3
  Mux2 : Mux  Inputs=3
  iniBODYAngles wrtVEH [rad] : Constant  Value=Roll0  SampleTime=TimeStep
  iniBODYAngles wrtVEH [rad]1 : Constant  Value=Pitch0  SampleTime=TimeStep
  iniVEHAngles wrtGLOB [rad] : Constant  Value=Yaw0  SampleTime=TimeStep
  iniVEHposition wrtGLOB [m] : Constant  Value=x0  SampleTime=TimeStep
  iniVEHposition wrtGLOB [m]1 : Constant  Value=y0  SampleTime=TimeStep
  iniVEHposition wrtGLOB [m]2 : Constant  Value=z0  SampleTime=TimeStep
  state2FullState : PreScanSimulinkLibrary/state2FullState  SystemSampleTime=-1
  StateBus : Outport  OutDataTypeStr=Bus: PRESCAN_STATEACTUATORDATA
  wires:
  Mux2/1 -> state2FullState/4
  iniVEHAngles wrtGLOB [rad]/1 -> Mux2/3
  Mux1/1 -> state2FullState/3
  Constant/1 -> Mux2/1, Mux2/2, Mux1/3
  iniBODYAngles wrtVEH [rad]1/1 -> Mux1/2
  iniBODYAngles wrtVEH [rad]/1 -> Mux1/1
  Mux/1 -> state2FullState/2
  iniVEHposition wrtGLOB [m]2/1 -> Mux/3
  iniVEHposition wrtGLOB [m]/1 -> Mux/1
  iniVEHposition wrtGLOB [m]1/1 -> Mux/2
  Demux/15 -> Bus Creator/15  "AngularVelocityYaw"
  Demux/14 -> Bus Creator/14  "AngularVelocityPitch"
  Demux/13 -> Bus Creator/13  "AngularVelocityRoll"
  Demux/12 -> Bus Creator/12  "OrientationYaw"
  Demux/11 -> Bus Creator/11  "OrientationPitch"
  Demux/10 -> Bus Creator/10  "OrientationRoll"
  Demux/9 -> Bus Creator/9  "AccelerationZ"
  Demux/8 -> Bus Creator/8  "AccelerationY"
  Demux/7 -> Bus Creator/7  "AccelerationX"
  Demux/6 -> Bus Creator/6  "VelocityZ"
  Demux/5 -> Bus Creator/5  "VelocityY"
  Demux/4 -> Bus Creator/4  "VelocityX"
  Demux/3 -> Bus Creator/3  "PositionZ"
  Demux/2 -> Bus Creator/2  "PositionY"
  Demux/1 -> Bus Creator/1  "PositionX"
  state2FullState/1 -> Demux/1
  State/1 -> state2FullState/1
  Bus Creator/1 -> StateBus/1

== system TL1_cs/BMW_X5_SUV_1/SELF_Demux/compas converter ==
  rotz [rad] : Inport
  cart2compas : Subsystem
  rad2deg : Gain  Gain=180/pi
  heading [deg] : Outport
  wires:
  rad2deg/1 -> cart2compas/1(Angle [deg])
  rotz [rad]/1 -> rad2deg/1
  cart2compas/1(heading [deg]) -> heading [deg]/1

== system TL1_cs/BMW_X5_SUV_1/Subsystem/Rotate over Z ==
  In1 : Inport
  In2 : Inport  Port=2
  In3 : Inport  Port=3
  Add : Sum  Inputs=+-
  Add1 : Sum
  Degrees to Radians1 : simulink_extras/Transformations/Degrees to Radians
  Product{,1..3} (4 alike) : Product
  Trigonometric Function : Trigonometry
  Trigonometric Function1 : Trigonometry  Operator=cos
  Out1 : Outport
  Out2 : Outport  Port=2
  wires:
  In2/1 -> Product/2, Product2/2
  Product/1 -> Add/1
  Trigonometric Function/1 -> Product2/1, Product1/1
  Trigonometric Function1/1 -> Product/1, Product3/1
  Degrees to Radians1/1 -> Trigonometric Function1/1, Trigonometric Function/1
  Product3/1 -> Add1/2
  Add1/1 -> Out2/1
  Product1/1 -> Add/2
  Product2/1 -> Add1/1
  In3/1 -> Product3/2, Product1/2
  In1/1 -> Degrees to Radians1/1
  Add/1 -> Out1/1

== system TL1_cs/BMW_X5_SUV_1/Subsystem/Spherical to cartesian ==
  In1 : Inport
  In2 : Inport  Port=2
  In3 : Inport  Port=3
  Constant : Constant  Value=-1  OutDataTypeStr=Inherit: Inherit via back propagation
  Product : Product
  Product1 : Product  Inputs=3
  Product2 : Product  Inputs=3
  Product3 : Product
  Trigonometric Function : Trigonometry  Operator=cos
  Trigonometric Function1 : Trigonometry
  Trigonometric Function2 : Trigonometry  Operator=cos
  Trigonometric Function3 : Trigonometry
  Out1 : Outport
  Out2 : Outport  Port=2
  Out3 : Outport  Port=3
  wires:
  In1/1 -> Product2/1, Product/1, Product1/1
  Product/1 -> Out3/1
  Product1/1 -> Out1/1
  Product2/1 -> Product3/1
  Trigonometric Function3/1 -> Product2/3
  Trigonometric Function2/1 -> Product1/3
  Trigonometric Function1/1 -> Product/2
  Trigonometric Function/1 -> Product1/2, Product2/2
  Constant/1 -> Product3/2
  Product3/1 -> Out2/1
  In3/1 -> Trigonometric Function1/1, Trigonometric Function/1
  In2/1 -> Trigonometric Function3/1, Trigonometric Function2/1

== system TL1_cs/BMW_X5_SUV_1/Subsystem1/Rotate over Z ==
  In1 : Inport
  In2 : Inport  Port=2
  In3 : Inport  Port=3
  Add : Sum  Inputs=+-
  Add1 : Sum
  Degrees to Radians1 : simulink_extras/Transformations/Degrees to Radians
  Product{,1..3} (4 alike) : Product
  Trigonometric Function : Trigonometry
  Trigonometric Function1 : Trigonometry  Operator=cos
  Out1 : Outport
  Out2 : Outport  Port=2
  wires:
  In2/1 -> Product/2, Product2/2
  Product/1 -> Add/1
  Trigonometric Function/1 -> Product2/1, Product1/1
  Trigonometric Function1/1 -> Product/1, Product3/1
  Degrees to Radians1/1 -> Trigonometric Function1/1, Trigonometric Function/1
  Product3/1 -> Add1/2
  Add1/1 -> Out2/1
  Product1/1 -> Add/2
  Product2/1 -> Add1/1
  In3/1 -> Product3/2, Product1/2
  In1/1 -> Degrees to Radians1/1
  Add/1 -> Out1/1

== system TL1_cs/BMW_X5_SUV_1/Subsystem1/Spherical to cartesian ==
  In1 : Inport
  In2 : Inport  Port=2
  In3 : Inport  Port=3
  Constant : Constant  Value=-1  OutDataTypeStr=Inherit: Inherit via back propagation
  Product : Product
  Product1 : Product  Inputs=3
  Product2 : Product  Inputs=3
  Product3 : Product
  Trigonometric Function : Trigonometry  Operator=cos
  Trigonometric Function1 : Trigonometry
  Trigonometric Function2 : Trigonometry  Operator=cos
  Trigonometric Function3 : Trigonometry
  Out1 : Outport
  Out2 : Outport  Port=2
  Out3 : Outport  Port=3
  wires:
  In1/1 -> Product2/1, Product/1, Product1/1
  Product/1 -> Out3/1
  Product1/1 -> Out1/1
  Product2/1 -> Product3/1
  Trigonometric Function3/1 -> Product2/3
  Trigonometric Function2/1 -> Product1/3
  Trigonometric Function1/1 -> Product/2
  Trigonometric Function/1 -> Product1/2, Product2/2
  Constant/1 -> Product3/2
  Product3/1 -> Out2/1
  In3/1 -> Trigonometric Function1/1, Trigonometric Function/1
  In2/1 -> Trigonometric Function3/1, Trigonometric Function2/1

== system TL1_cs/BMW_X5_SUV_1/Subsystem2/Rotate over Z ==
  In1 : Inport
  In2 : Inport  Port=2
  In3 : Inport  Port=3
  Add : Sum  Inputs=+-
  Add1 : Sum
  Degrees to Radians1 : simulink_extras/Transformations/Degrees to Radians
  Product{,1..3} (4 alike) : Product
  Trigonometric Function : Trigonometry
  Trigonometric Function1 : Trigonometry  Operator=cos
  Out1 : Outport
  Out2 : Outport  Port=2
  wires:
  In2/1 -> Product/2, Product2/2
  Product/1 -> Add/1
  Trigonometric Function/1 -> Product2/1, Product1/1
  Trigonometric Function1/1 -> Product/1, Product3/1
  Degrees to Radians1/1 -> Trigonometric Function1/1, Trigonometric Function/1
  Product3/1 -> Add1/2
  Add1/1 -> Out2/1
  Product1/1 -> Add/2
  Product2/1 -> Add1/1
  In3/1 -> Product3/2, Product1/2
  In1/1 -> Degrees to Radians1/1
  Add/1 -> Out1/1

== system TL1_cs/BMW_X5_SUV_1/Subsystem2/Spherical to cartesian ==
  In1 : Inport
  In2 : Inport  Port=2
  In3 : Inport  Port=3
  Constant : Constant  Value=-1  OutDataTypeStr=Inherit: Inherit via back propagation
  Product : Product
  Product1 : Product  Inputs=3
  Product2 : Product  Inputs=3
  Product3 : Product
  Trigonometric Function : Trigonometry  Operator=cos
  Trigonometric Function1 : Trigonometry
  Trigonometric Function2 : Trigonometry  Operator=cos
  Trigonometric Function3 : Trigonometry
  Out1 : Outport
  Out2 : Outport  Port=2
  Out3 : Outport  Port=3
  wires:
  In1/1 -> Product2/1, Product/1, Product1/1
  Product/1 -> Out3/1
  Product1/1 -> Out1/1
  Product2/1 -> Product3/1
  Trigonometric Function3/1 -> Product2/3
  Trigonometric Function2/1 -> Product1/3
  Trigonometric Function1/1 -> Product/2
  Trigonometric Function/1 -> Product1/2, Product2/2
  Constant/1 -> Product3/2
  Product3/1 -> Out2/1
  In3/1 -> Trigonometric Function1/1, Trigonometric Function/1
  In2/1 -> Trigonometric Function3/1, Trigonometric Function2/1

== system TL1_cs/BMW_X5_SUV_1/Subsystem3/Rotate over Z ==
  In1 : Inport
  In2 : Inport  Port=2
  In3 : Inport  Port=3
  Add : Sum  Inputs=+-
  Add1 : Sum
  Degrees to Radians1 : simulink_extras/Transformations/Degrees to Radians
  Product{,1..3} (4 alike) : Product
  Trigonometric Function : Trigonometry
  Trigonometric Function1 : Trigonometry  Operator=cos
  Out1 : Outport
  Out2 : Outport  Port=2
  wires:
  In2/1 -> Product/2, Product2/2
  Product/1 -> Add/1
  Trigonometric Function/1 -> Product2/1, Product1/1
  Trigonometric Function1/1 -> Product/1, Product3/1
  Degrees to Radians1/1 -> Trigonometric Function1/1, Trigonometric Function/1
  Product3/1 -> Add1/2
  Add1/1 -> Out2/1
  Product1/1 -> Add/2
  Product2/1 -> Add1/1
  In3/1 -> Product3/2, Product1/2
  In1/1 -> Degrees to Radians1/1
  Add/1 -> Out1/1

== system TL1_cs/BMW_X5_SUV_1/Subsystem3/Spherical to cartesian ==
  In1 : Inport
  In2 : Inport  Port=2
  In3 : Inport  Port=3
  Constant : Constant  Value=-1  OutDataTypeStr=Inherit: Inherit via back propagation
  Product : Product
  Product1 : Product  Inputs=3
  Product2 : Product  Inputs=3
  Product3 : Product
  Trigonometric Function : Trigonometry  Operator=cos
  Trigonometric Function1 : Trigonometry
  Trigonometric Function2 : Trigonometry  Operator=cos
  Trigonometric Function3 : Trigonometry
  Out1 : Outport
  Out2 : Outport  Port=2
  Out3 : Outport  Port=3
  wires:
  In1/1 -> Product2/1, Product/1, Product1/1
  Product/1 -> Out3/1
  Product1/1 -> Out1/1
  Product2/1 -> Product3/1
  Trigonometric Function3/1 -> Product2/3
  Trigonometric Function2/1 -> Product1/3
  Trigonometric Function1/1 -> Product/2
  Trigonometric Function/1 -> Product1/2, Product2/2
  Constant/1 -> Product3/2
  Product3/1 -> Out2/1
  In3/1 -> Trigonometric Function1/1, Trigonometric Function/1
  In2/1 -> Trigonometric Function3/1, Trigonometric Function2/1

== system TL1_cs/Ford_Fiesta_Hatchback_1/AIR_1_Demux/Activate_Switch ==
  BeamID : Inport
  Heading : Inport  Port=2
  Constant : Constant  Value=0
  Product1 : Product  RndMeth=Zero
  Relational Operator : RelationalOperator  Operator=~=  OutDataTypeStr=boolean  RndMeth=Nearest
  On/Off : Outport
  wires:
  Constant/1 -> Relational Operator/1
  Relational Operator/1 -> Product1/1
  BeamID/1 -> Relational Operator/2
  Product1/1 -> On/Off/1
  Heading/1 -> Product1/2

== system TL1_cs/Ford_Fiesta_Hatchback_1/AIR_1_Demux/Signal2ArrayOfSignals1 ==
  note: Set mask parameter VECTORLENGTH
      |  to MAXMESSAGES
  note: Initial state of Previous vector block
      | set to zeros(VECTORLENGTH,1)
  LoopIndex : Inport
  Element : Inport  Port=2
  Assignment : Assignment  IndexOptions=Index vector (port)  Indices=1  OutputSizes=1
  Previous vector : Memory  InitialCondition=zeros(VECTORLENGTH,1)  InheritSampleTime=on
  ArrayofElements : Outport
  wires:
  Element/1 -> Assignment/2
  LoopIndex/1 -> Assignment/3
  Previous vector/1 -> Assignment/1
  Assignment/1 -> ArrayofElements/1, Previous vector/1

== system TL1_cs/Ford_Fiesta_Hatchback_1/AIR_1_Demux/Signal2ArrayOfSignals2 ==
  note: Set mask parameter VECTORLENGTH
      |  to MAXMESSAGES
  note: Initial state of Previous vector block
      | set to zeros(VECTORLENGTH,1)
  LoopIndex : Inport
  Element : Inport  Port=2
  Assignment : Assignment  IndexOptions=Index vector (port)  Indices=1  OutputSizes=1
  Previous vector : Memory  InitialCondition=zeros(VECTORLENGTH,1)  InheritSampleTime=on
  ArrayofElements : Outport
  wires:
  Element/1 -> Assignment/2
  LoopIndex/1 -> Assignment/3
  Previous vector/1 -> Assignment/1
  Assignment/1 -> ArrayofElements/1, Previous vector/1

== system TL1_cs/Ford_Fiesta_Hatchback_1/AIR_1_Demux/Signal2ArrayOfSignals3 ==
  note: Set mask parameter VECTORLENGTH
      |  to MAXMESSAGES
  note: Initial state of Previous vector block
      | set to zeros(VECTORLENGTH,1)
  LoopIndex : Inport
  Element : Inport  Port=2
  Assignment : Assignment  IndexOptions=Index vector (port)  Indices=1  OutputSizes=1
  Previous vector : Memory  InitialCondition=zeros(VECTORLENGTH,1)  InheritSampleTime=on
  ArrayofElements : Outport
  wires:
  Element/1 -> Assignment/2
  LoopIndex/1 -> Assignment/3
  Previous vector/1 -> Assignment/1
  Assignment/1 -> ArrayofElements/1, Previous vector/1

== system TL1_cs/Ford_Fiesta_Hatchback_1/AIR_1_Demux/Signal2ArrayOfSignals4 ==
  note: Set mask parameter VECTORLENGTH
      |  to MAXMESSAGES
  note: Initial state of Previous vector block
      | set to zeros(VECTORLENGTH,1)
  LoopIndex : Inport
  Element : Inport  Port=2
  Assignment : Assignment  IndexOptions=Index vector (port)  Indices=1  OutputSizes=1
  Previous vector : Memory  InitialCondition=zeros(VECTORLENGTH,1)  InheritSampleTime=on
  ArrayofElements : Outport
  wires:
  Element/1 -> Assignment/2
  LoopIndex/1 -> Assignment/3
  Previous vector/1 -> Assignment/1
  Assignment/1 -> ArrayofElements/1, Previous vector/1
